simulink model "task1"  (R2016b)
settings: Solver=VariableStepAuto  StartTime=0.0  StopTime=10.0  RelTol=1e-3
libraries: commutil2 x1
settings Model: Creator=zhangjin  LastModifiedBy=zhangjin

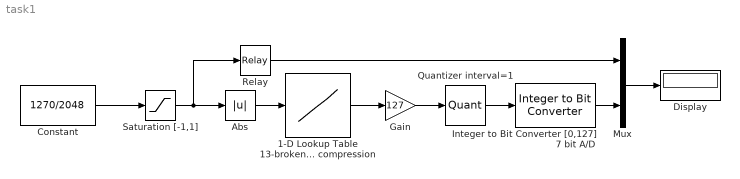
== system task1 ==
  1-D Lookup Table 13-broken line compression : Lookup_n-D  NumberOfTableDimensions=1  BreakpointsForDimension1=[-5:5]  Table=tanh([-5:5])  InternalRulePriority=Speed  RndMeth=Simplest  InputSameDT=on
  Abs : Abs
  Constant : Constant  Value=1270/2048
  Display : Display
  Gain : Gain  Gain=127
  Integer to Bit Converter [0,127] 7 bit A/D : commutil2/Integer to Bit Converter  nbits=3  signedInputValues=Unsigned  bitOrder=MSB first  outDtype=Inherit via internal rule
  Mux : Mux  Inputs=2
  Quantizer interval=1 : Quantizer  QuantizationInterval=1  LinearizeAsGain=off
  Relay : Relay
  Saturation [-1,1] : Saturate  UpperLimit=1  LowerLimit=-1
  wires:
  Constant/1 -> Saturation [-1,1]/1
  Saturation [-1,1]/1 -> Relay/1, Abs/1
  Abs/1 -> 1-D Lookup Table 13-broken line compression/1
  1-D Lookup Table 13-broken line compression/1 -> Gain/1
  Gain/1 -> Quantizer interval=1/1
  Quantizer interval=1/1 -> Integer to Bit Converter [0,127] 7 bit A/D/1
  Integer to Bit Converter [0,127] 7 bit A/D/1 -> Mux/2
  Relay/1 -> Mux/1
  Mux/1 -> Display/1
